simulink model "case6"  (R2024b)
settings: Solver=FixedStepAuto  StartTime=0  StopTime=1  FixedStep=1e-7  RelTol=1e-3
values from neighbouring files (symbols this model uses):
  SG_D_1_D = 0.01056    [IEEE9_case_parameters.m]    (also in case1_parameters.m; case2_parameters.m; case3_parameters.m; case4_parameters.m)
  SG_D_1_EnableSaturation = 0    [IEEE9_case_parameters.m]    (also in case1_parameters.m; case2_parameters.m; case3_parameters.m; case4_parameters.m)
  SG_D_1_f0 = 60    [IEEE9_case_parameters.m]    (also in case1_parameters.m; case2_parameters.m; case3_parameters.m; case4_parameters.m)
  SG_D_1_H = 7.5    [IEEE9_case_parameters.m]    (also in case1_parameters.m; case2_parameters.m; case3_parameters.m; case4_parameters.m)
  SG_D_1_K_A = 20    [IEEE9_case_parameters.m]    (also in case1_parameters.m; case2_parameters.m; case3_parameters.m; case4_parameters.m)
  SG_D_1_K_E = 1.000000e+1    (= 10)    [IEEE9_case_parameters.m]    (also in case1_parameters.m; case2_parameters.m; case3_parameters.m; case4_parameters.m)
  SG_D_1_K_F = 2.363    [IEEE9_case_parameters.m]    (also in case1_parameters.m; case2_parameters.m; case3_parameters.m; case4_parameters.m)
  SG_D_1_K_s = 0.5    [IEEE9_case_parameters.m]    (also in case1_parameters.m = 5; case2_parameters.m = 5; case3_parameters.m = 5; case4_parameters.m = 5)
  SG_D_1_R_a = 0.001088    [IEEE9_case_parameters.m]    (also in case1_parameters.m; case2_parameters.m; case3_parameters.m; case4_parameters.m)
  SG_D_1_S_A = 1    [IEEE9_case_parameters.m]    (also in case1_parameters.m; case2_parameters.m; case3_parameters.m; case4_parameters.m)
  SG_D_1_S_B = 0.103    [IEEE9_case_parameters.m]    (also in case1_parameters.m; case2_parameters.m; case3_parameters.m; case4_parameters.m)
  SG_D_1_S_N = 10.659857    [IEEE9_case_parameters.m]    (also in case1_parameters.m; case2_parameters.m; case3_parameters.m; case4_parameters.m)
  SG_D_1_SpeedPara = 200    [IEEE9_case_parameters.m]    (also in case1_parameters.m; case2_parameters.m; case3_parameters.m; case4_parameters.m)
  SG_D_1_T_0 = 0.720173    [IEEE9_case_parameters.m]    (also in case1_parameters.m = 0.755522; case2_parameters.m = 0.808931; case3_parameters.m = 0.869402; case4_parameters.m = 0.729316)
  SG_D_1_T_1 = 0.3    [IEEE9_case_parameters.m]    (also in case1_parameters.m; case2_parameters.m; case3_parameters.m; case4_parameters.m)
  SG_D_1_T_2 = 0.05    [IEEE9_case_parameters.m]    (also in case1_parameters.m; case2_parameters.m; case3_parameters.m; case4_parameters.m)
  SG_D_1_T_3 = 0.02    [IEEE9_case_parameters.m]    (also in case1_parameters.m; case2_parameters.m; case3_parameters.m; case4_parameters.m)
  SG_D_1_T_4 = 0.005    [IEEE9_case_parameters.m]    (also in case1_parameters.m; case2_parameters.m; case3_parameters.m; case4_parameters.m)
  SG_D_1_T_A = 0.02    [IEEE9_case_parameters.m]    (also in case1_parameters.m; case2_parameters.m; case3_parameters.m; case4_parameters.m)
  SG_D_1_T_dd = 8.000000e+0    (= 8)    [IEEE9_case_parameters.m]    (also in case1_parameters.m; case2_parameters.m; case3_parameters.m; case4_parameters.m)
  SG_D_1_T_ddd = 0.04    [IEEE9_case_parameters.m]    (also in case1_parameters.m; case2_parameters.m; case3_parameters.m; case4_parameters.m)
  SG_D_1_T_E = 0.314    [IEEE9_case_parameters.m]    (also in case1_parameters.m; case2_parameters.m; case3_parameters.m; case4_parameters.m)
  SG_D_1_T_F = 0.35    [IEEE9_case_parameters.m]    (also in case1_parameters.m; case2_parameters.m; case3_parameters.m; case4_parameters.m)
  SG_D_1_T_qd = 0.8    [IEEE9_case_parameters.m]    (also in case1_parameters.m; case2_parameters.m; case3_parameters.m; case4_parameters.m)
  SG_D_1_T_qdd = 0.02    [IEEE9_case_parameters.m]    (also in case1_parameters.m; case2_parameters.m; case3_parameters.m; case4_parameters.m)
  SG_D_1_T_speed = 0.1    [IEEE9_case_parameters.m]    (also in case1_parameters.m = 200; case2_parameters.m = 200; case3_parameters.m = 200; case4_parameters.m = 200)
  SG_D_1_T_w = 0.5    [IEEE9_case_parameters.m]    (also in case1_parameters.m; case2_parameters.m; case3_parameters.m; case4_parameters.m)
  SG_D_1_V_ref = 1.990276    [IEEE9_case_parameters.m]    (also in case1_parameters.m = 2.042296; case2_parameters.m = 2.051388; case3_parameters.m = 2.089584; case4_parameters.m = 2.01845)
  SG_D_1_w_ref = 376.991118    [IEEE9_case_parameters.m]    (also in case1_parameters.m; case2_parameters.m; case3_parameters.m; case4_parameters.m)
  SG_D_1_wb = 6.000000e+1    (= 60)    [IEEE9_case_parameters.m]    (also in case1_parameters.m; case2_parameters.m; case3_parameters.m; case4_parameters.m)
  SG_D_1_x_d = 1.9    [IEEE9_case_parameters.m]    (also in case1_parameters.m; case2_parameters.m; case3_parameters.m; case4_parameters.m)
  SG_D_1_x_dd = 0.302    [IEEE9_case_parameters.m]    (also in case1_parameters.m; case2_parameters.m; case3_parameters.m; case4_parameters.m)
  SG_D_1_x_ddd = 0.204    [IEEE9_case_parameters.m]    (also in case1_parameters.m; case2_parameters.m; case3_parameters.m; case4_parameters.m)
  SG_D_1_x_l = 0.05    [IEEE9_case_parameters.m]    (also in case1_parameters.m; case2_parameters.m; case3_parameters.m; case4_parameters.m)
  SG_D_1_x_q = 1.3    [IEEE9_case_parameters.m]    (also in case1_parameters.m; case2_parameters.m; case3_parameters.m; case4_parameters.m)
  SG_D_1_x_qd = 0.5    [IEEE9_case_parameters.m]    (also in case1_parameters.m; case2_parameters.m; case3_parameters.m; case4_parameters.m)
  SG_D_1_x_qdd = 0.3    [IEEE9_case_parameters.m]    (also in case1_parameters.m; case2_parameters.m; case3_parameters.m; case4_parameters.m)
  SG_D_2_D = 0.02    [IEEE9_case_parameters.m]    (also in case1_parameters.m; case2_parameters.m; case3_parameters.m; case4_parameters.m)
  SG_D_2_EnableSaturation = 0    [IEEE9_case_parameters.m]    (also in case1_parameters.m; case2_parameters.m; case3_parameters.m; case4_parameters.m)
  SG_D_2_f0 = 60    [IEEE9_case_parameters.m]    (also in case1_parameters.m; case2_parameters.m; case3_parameters.m; case4_parameters.m)
  SG_D_2_H = 8.000000e+0    (= 8)    [IEEE9_case_parameters.m]    (also in case1_parameters.m; case2_parameters.m; case3_parameters.m; case4_parameters.m)
  SG_D_2_K_A = 20    [IEEE9_case_parameters.m]    (also in case1_parameters.m; case2_parameters.m; case3_parameters.m; case4_parameters.m)
  SG_D_2_K_E = 1.000000e+1    (= 10)    [IEEE9_case_parameters.m]    (also in case1_parameters.m; case2_parameters.m; case3_parameters.m; case4_parameters.m)
  SG_D_2_K_F = 2.363    [IEEE9_case_parameters.m]    (also in case1_parameters.m; case2_parameters.m; case3_parameters.m; case4_parameters.m)
  SG_D_2_K_s = 0.5    [IEEE9_case_parameters.m]    (also in case1_parameters.m = 4; case2_parameters.m = 4; case3_parameters.m = 4; case4_parameters.m = 4)
  SG_D_2_R_a = 0.001088    [IEEE9_case_parameters.m]    (also in case1_parameters.m; case2_parameters.m; case3_parameters.m; case4_parameters.m)
  SG_D_2_S_A = 1    [IEEE9_case_parameters.m]    (also in case1_parameters.m; case2_parameters.m; case3_parameters.m; case4_parameters.m)
  SG_D_2_S_B = 0.103    [IEEE9_case_parameters.m]    (also in case1_parameters.m; case2_parameters.m; case3_parameters.m; case4_parameters.m)
  SG_D_2_S_N = 10.659857    [IEEE9_case_parameters.m]    (also in case1_parameters.m; case2_parameters.m; case3_parameters.m; case4_parameters.m)
  SG_D_2_SpeedPara = 200    [IEEE9_case_parameters.m]    (also in case1_parameters.m; case2_parameters.m; case3_parameters.m; case4_parameters.m)
  SG_D_2_T_0 = 1.632913    [IEEE9_case_parameters.m]    (also in case1_parameters.m = 1.632925; case2_parameters.m = 1.632915; case3_parameters.m = 1.632914; case4_parameters.m = 1.632927)
  SG_D_2_T_1 = 0.2    [IEEE9_case_parameters.m]    (also in case1_parameters.m; case2_parameters.m; case3_parameters.m; case4_parameters.m)
  SG_D_2_T_2 = 0.05    [IEEE9_case_parameters.m]    (also in case1_parameters.m; case2_parameters.m; case3_parameters.m; case4_parameters.m)
  SG_D_2_T_3 = 0.02    [IEEE9_case_parameters.m]    (also in case1_parameters.m; case2_parameters.m; case3_parameters.m; case4_parameters.m)
  SG_D_2_T_4 = 0.005    [IEEE9_case_parameters.m]    (also in case1_parameters.m; case2_parameters.m; case3_parameters.m; case4_parameters.m)
  SG_D_2_T_A = 0.02    [IEEE9_case_parameters.m]    (also in case1_parameters.m; case2_parameters.m; case3_parameters.m; case4_parameters.m)
  SG_D_2_T_dd = 7.9    [IEEE9_case_parameters.m]    (also in case1_parameters.m; case2_parameters.m; case3_parameters.m; case4_parameters.m)
  SG_D_2_T_ddd = 0.04    [IEEE9_case_parameters.m]    (also in case1_parameters.m; case2_parameters.m; case3_parameters.m; case4_parameters.m)
  SG_D_2_T_E = 0.314    [IEEE9_case_parameters.m]    (also in case1_parameters.m; case2_parameters.m; case3_parameters.m; case4_parameters.m)
  SG_D_2_T_F = 0.35    [IEEE9_case_parameters.m]    (also in case1_parameters.m; case2_parameters.m; case3_parameters.m; case4_parameters.m)
  SG_D_2_T_qd = 0.8    [IEEE9_case_parameters.m]    (also in case1_parameters.m; case2_parameters.m; case3_parameters.m; case4_parameters.m)
  SG_D_2_T_qdd = 0.015    [IEEE9_case_parameters.m]    (also in case1_parameters.m; case2_parameters.m; case3_parameters.m; case4_parameters.m)
  SG_D_2_T_speed = 0.1    [IEEE9_case_parameters.m]    (also in case1_parameters.m = 150; case2_parameters.m = 150; case3_parameters.m = 150; case4_parameters.m = 150)
  SG_D_2_T_w = 0.35    [IEEE9_case_parameters.m]    (also in case1_parameters.m; case2_parameters.m; case3_parameters.m; case4_parameters.m)
  SG_D_2_V_ref = 2.58547    [IEEE9_case_parameters.m]    (also in case1_parameters.m = 2.597896; case2_parameters.m = 2.587136; case3_parameters.m = 2.586042; case4_parameters.m = 2.599679)
  SG_D_2_w_ref = 376.991118    [IEEE9_case_parameters.m]    (also in case1_parameters.m; case2_parameters.m; case3_parameters.m; case4_parameters.m)
  SG_D_2_wb = 6.000000e+1    (= 60)    [IEEE9_case_parameters.m]    (also in case1_parameters.m; case2_parameters.m; case3_parameters.m; case4_parameters.m)
  SG_D_2_x_d = 1.8    [IEEE9_case_parameters.m]    (also in case1_parameters.m; case2_parameters.m; case3_parameters.m; case4_parameters.m)
  SG_D_2_x_dd = 0.302    [IEEE9_case_parameters.m]    (also in case1_parameters.m; case2_parameters.m; case3_parameters.m; case4_parameters.m)
  SG_D_2_x_ddd = 0.204    [IEEE9_case_parameters.m]    (also in case1_parameters.m; case2_parameters.m; case3_parameters.m; case4_parameters.m)
  SG_D_2_x_l = 0.05    [IEEE9_case_parameters.m]    (also in case1_parameters.m; case2_parameters.m; case3_parameters.m; case4_parameters.m)
  SG_D_2_x_q = 1.25    [IEEE9_case_parameters.m]    (also in case1_parameters.m; case2_parameters.m; case3_parameters.m; case4_parameters.m)
  SG_D_2_x_qd = 0.5    [IEEE9_case_parameters.m]    (also in case1_parameters.m; case2_parameters.m; case3_parameters.m; case4_parameters.m)
  SG_D_2_x_qdd = 0.3    [IEEE9_case_parameters.m]    (also in case1_parameters.m; case2_parameters.m; case3_parameters.m; case4_parameters.m)
  SG_D_3_D = 0.02    [IEEE9_case_parameters.m]    (also in case1_parameters.m; case2_parameters.m; case3_parameters.m; case4_parameters.m)
  SG_D_3_EnableSaturation = 0    [IEEE9_case_parameters.m]    (also in case1_parameters.m; case2_parameters.m; case3_parameters.m; case4_parameters.m)
  SG_D_3_f0 = 60    [IEEE9_case_parameters.m]    (also in case1_parameters.m; case2_parameters.m; case3_parameters.m; case4_parameters.m)
  SG_D_3_H = 7.7    [IEEE9_case_parameters.m]    (also in case1_parameters.m; case2_parameters.m; case3_parameters.m; case4_parameters.m)
  SG_D_3_K_A = 20    [IEEE9_case_parameters.m]    (also in case1_parameters.m; case2_parameters.m; case3_parameters.m; case4_parameters.m)
  SG_D_3_K_E = 1.000000e+1    (= 10)    [IEEE9_case_parameters.m]    (also in case1_parameters.m; case2_parameters.m; case3_parameters.m; case4_parameters.m)
  SG_D_3_K_F = 2.363    [IEEE9_case_parameters.m]    (also in case1_parameters.m; case2_parameters.m; case3_parameters.m; case4_parameters.m)
  SG_D_3_K_s = 0.2    [IEEE9_case_parameters.m]    (also in case1_parameters.m = 2; case2_parameters.m = 2; case3_parameters.m = 2; case4_parameters.m = 2)
  SG_D_3_R_a = 0.001088    [IEEE9_case_parameters.m]    (also in case1_parameters.m; case2_parameters.m; case3_parameters.m; case4_parameters.m)
  SG_D_3_S_A = 1    [IEEE9_case_parameters.m]    (also in case1_parameters.m; case2_parameters.m; case3_parameters.m; case4_parameters.m)
  SG_D_3_S_B = 0.103    [IEEE9_case_parameters.m]    (also in case1_parameters.m; case2_parameters.m; case3_parameters.m; case4_parameters.m)
  SG_D_3_S_N = 10.659857    [IEEE9_case_parameters.m]    (also in case1_parameters.m; case2_parameters.m; case3_parameters.m; case4_parameters.m)
  SG_D_3_SpeedPara = 200    [IEEE9_case_parameters.m]    (also in case1_parameters.m; case2_parameters.m; case3_parameters.m; case4_parameters.m)
  SG_D_3_T_0 = 0.850788    [IEEE9_case_parameters.m]    (also in case1_parameters.m = 0.850786; case2_parameters.m = 0.850787; case3_parameters.m; case4_parameters.m = 0.850786)
  SG_D_3_T_1 = 0.2    [IEEE9_case_parameters.m]    (also in case1_parameters.m; case2_parameters.m; case3_parameters.m; case4_parameters.m)
  SG_D_3_T_2 = 0.05    [IEEE9_case_parameters.m]    (also in case1_parameters.m; case2_parameters.m; case3_parameters.m; case4_parameters.m)
  SG_D_3_T_3 = 0.02    [IEEE9_case_parameters.m]    (also in case1_parameters.m; case2_parameters.m; case3_parameters.m; case4_parameters.m)
  SG_D_3_T_4 = 0.005    [IEEE9_case_parameters.m]    (also in case1_parameters.m; case2_parameters.m; case3_parameters.m; case4_parameters.m)
  SG_D_3_T_A = 0.02    [IEEE9_case_parameters.m]    (also in case1_parameters.m; case2_parameters.m; case3_parameters.m; case4_parameters.m)
  SG_D_3_T_dd = 8.1    [IEEE9_case_parameters.m]    (also in case1_parameters.m; case2_parameters.m; case3_parameters.m; case4_parameters.m)
  SG_D_3_T_ddd = 0.04    [IEEE9_case_parameters.m]    (also in case1_parameters.m; case2_parameters.m; case3_parameters.m; case4_parameters.m)
  SG_D_3_T_E = 0.314    [IEEE9_case_parameters.m]    (also in case1_parameters.m; case2_parameters.m; case3_parameters.m; case4_parameters.m)
  SG_D_3_T_F = 0.35    [IEEE9_case_parameters.m]    (also in case1_parameters.m; case2_parameters.m; case3_parameters.m; case4_parameters.m)
  SG_D_3_T_qd = 0.8    [IEEE9_case_parameters.m]    (also in case1_parameters.m; case2_parameters.m; case3_parameters.m; case4_parameters.m)
  SG_D_3_T_qdd = 0.015    [IEEE9_case_parameters.m]    (also in case1_parameters.m; case2_parameters.m; case3_parameters.m; case4_parameters.m)
  SG_D_3_T_speed = 0.1    [IEEE9_case_parameters.m]    (also in case1_parameters.m = 180; case2_parameters.m = 180; case3_parameters.m = 180; case4_parameters.m = 180)
  SG_D_3_T_w = 0.4    [IEEE9_case_parameters.m]    (also in case1_parameters.m; case2_parameters.m; case3_parameters.m; case4_parameters.m)
  SG_D_3_V_ref = 1.892727    [IEEE9_case_parameters.m]    (also in case1_parameters.m = 1.906439; case2_parameters.m = 1.895535; case3_parameters.m = 1.892105; case4_parameters.m = 1.906598)
  SG_D_3_w_ref = 376.991118    [IEEE9_case_parameters.m]    (also in case1_parameters.m; case2_parameters.m; case3_parameters.m; case4_parameters.m)
  SG_D_3_wb = 6.000000e+1    (= 60)    [IEEE9_case_parameters.m]    (also in case1_parameters.m; case2_parameters.m; case3_parameters.m; case4_parameters.m)
  SG_D_3_x_d = 1.85    [IEEE9_case_parameters.m]    (also in case1_parameters.m; case2_parameters.m; case3_parameters.m; case4_parameters.m)
  SG_D_3_x_dd = 0.302    [IEEE9_case_parameters.m]    (also in case1_parameters.m; case2_parameters.m; case3_parameters.m; case4_parameters.m)
  SG_D_3_x_ddd = 0.204    [IEEE9_case_parameters.m]    (also in case1_parameters.m; case2_parameters.m; case3_parameters.m; case4_parameters.m)
  SG_D_3_x_l = 0.05    [IEEE9_case_parameters.m]    (also in case1_parameters.m; case2_parameters.m; case3_parameters.m; case4_parameters.m)
  SG_D_3_x_q = 1.2    [IEEE9_case_parameters.m]    (also in case1_parameters.m; case2_parameters.m; case3_parameters.m; case4_parameters.m)
  SG_D_3_x_qd = 0.5    [IEEE9_case_parameters.m]    (also in case1_parameters.m; case2_parameters.m; case3_parameters.m; case4_parameters.m)
  SG_D_3_x_qdd = 0.3    [IEEE9_case_parameters.m]    (also in case1_parameters.m; case2_parameters.m; case3_parameters.m; case4_parameters.m)
(part 3 of 12)

== system case6/AC_1/d_id_load_7_block ==
  note: d_id_load_7 in case6
      | $376.991118430775\,\mathrm{iq}_{\mathrm{load},7}-1042.68025815291\,\mathrm{id}_{\mathrm{load},7}+1171.3449213978\,\mathrm{vd}_{\mathrm{bus},7}$
      | Automatically generated on 2025-10-31 19:20:41 .
  State_id_load_7_ed6d0 : Inport
  State_iq_load_7_25236 : Inport  Port=2
  State_vd_bus_7_f8e0f : Inport  Port=3
  Add_24cd1 : Sum
  Add_83972 : Sum
  Constant_-1042.68025815291_f7e22 : Constant  Value=-1042.68025815291
  Constant_1171.3449213978_b1cfa : Constant  Value=1171.3449213978
  Constant_376.991118430775_13427 : Constant  Value=376.991118430775
  Product_2e9ca : Product
  Product_abc47 : Product
  Product_b8994 : Product
  Blockout_d_id_load_7_4bf44 : Outport
  wires:
  Constant_-1042.68025815291_f7e22/1 -> Product_2e9ca/1
  Product_b8994/1 -> Add_83972/2
  State_id_load_7_ed6d0/1 -> Product_2e9ca/2
  Constant_376.991118430775_13427/1 -> Product_b8994/1
  Product_2e9ca/1 -> Add_83972/1
  State_iq_load_7_25236/1 -> Product_b8994/2
  Constant_1171.3449213978_b1cfa/1 -> Product_abc47/1
  State_vd_bus_7_f8e0f/1 -> Product_abc47/2
  Add_83972/1 -> Add_24cd1/1
  Product_abc47/1 -> Add_24cd1/2
  Add_24cd1/1 -> Blockout_d_id_load_7_4bf44/1

== system case6/AC_1/d_id_load_9_block ==
  note: d_id_load_9 in case6
      | $376.991118430775\,\mathrm{iq}_{\mathrm{load},9}-912.345225962008\,\mathrm{id}_{\mathrm{load},9}+1407.02236836831\,\mathrm{vd}_{\mathrm{bus},9}$
      | Automatically generated on 2025-10-31 19:20:44 .
  State_id_load_9_971b0 : Inport
  State_iq_load_9_63cda : Inport  Port=2
  State_vd_bus_9_1fdd2 : Inport  Port=3
  Add_11f24 : Sum
  Add_b37a4 : Sum
  Constant_-912.345225962008_b413d : Constant  Value=-912.345225962008
  Constant_1407.02236836831_5bcda : Constant  Value=1407.02236836831
  Constant_376.991118430775_b0d4f : Constant  Value=376.991118430775
  Product_84c17 : Product
  Product_90090 : Product
  Product_fc741 : Product
  Blockout_d_id_load_9_0a7d1 : Outport
  wires:
  Constant_-912.345225962008_b413d/1 -> Product_84c17/1
  Product_90090/1 -> Add_b37a4/2
  State_id_load_9_971b0/1 -> Product_84c17/2
  Constant_376.991118430775_b0d4f/1 -> Product_90090/1
  Product_84c17/1 -> Add_b37a4/1
  State_iq_load_9_63cda/1 -> Product_90090/2
  Constant_1407.02236836831_5bcda/1 -> Product_fc741/1
  State_vd_bus_9_1fdd2/1 -> Product_fc741/2
  Add_b37a4/1 -> Add_11f24/1
  Product_fc741/1 -> Add_11f24/2
  Add_11f24/1 -> Blockout_d_id_load_9_0a7d1/1

== system case6/AC_1/d_iq_line_1_4_block ==
  note: d_iq_line_1_4 in case6
      | $6868.34433494245\,\mathrm{vq}_{\mathrm{bus},1}-376.991118430775\,\mathrm{id}_{\mathrm{line},1,4}-6868.34433494245\,\mathrm{vq}_{\mathrm{bus},4}$
      | Automatically generated on 2025-10-31 19:20:48 .
  State_id_line_1_4_5a9b1 : Inport
  State_vq_bus_1_6b284 : Inport  Port=2
  State_vq_bus_4_deba6 : Inport  Port=3
  Add_c85ec : Sum
  Constant_-376.991118430775_bb66e : Constant  Value=-376.991118430775
  Constant_6868.34433494245_3906b : Constant  Value=6868.34433494245
  Constant_6868.34433494245_64567 : Constant  Value=6868.34433494245
  Product_0c770 : Product
  Product_838f3 : Product
  Product_8e35f : Product
  Subtract_df51f : Sum  Inputs=+-
  Blockout_d_iq_line_1_4_201af : Outport
  wires:
  Constant_-376.991118430775_bb66e/1 -> Product_0c770/1
  Product_8e35f/1 -> Add_c85ec/2
  State_id_line_1_4_5a9b1/1 -> Product_0c770/2
  Constant_6868.34433494245_3906b/1 -> Product_8e35f/1
  Product_0c770/1 -> Add_c85ec/1
  Subtract_df51f/1 -> Blockout_d_iq_line_1_4_201af/1
  State_vq_bus_1_6b284/1 -> Product_8e35f/2
  Constant_6868.34433494245_64567/1 -> Product_838f3/1
  State_vq_bus_4_deba6/1 -> Product_838f3/2
  Add_c85ec/1 -> Subtract_df51f/1
  Product_838f3/1 -> Subtract_df51f/2

== system case6/AC_1/d_iq_line_3_6_block ==
  note: d_iq_line_3_6 in case6
      | $6751.13709373183\,\mathrm{vq}_{\mathrm{bus},3}-376.991118430775\,\mathrm{id}_{\mathrm{line},3,6}-6751.13709373183\,\mathrm{vq}_{\mathrm{bus},6}$
      | Automatically generated on 2025-10-31 19:20:58 .
  State_id_line_3_6_29fbd : Inport
  State_vq_bus_3_8aa9d : Inport  Port=2
  State_vq_bus_6_e5847 : Inport  Port=3
  Add_bc3ba : Sum
  Constant_-376.991118430775_cf978 : Constant  Value=-376.991118430775
  Constant_6751.13709373183_457c0 : Constant  Value=6751.13709373183
  Constant_6751.13709373183_acfcf : Constant  Value=6751.13709373183
  Product_533ae : Product
  Product_6e6cb : Product
  Product_998dd : Product
  Subtract_d0816 : Sum  Inputs=+-
  Blockout_d_iq_line_3_6_a81a1 : Outport
  wires:
  Constant_-376.991118430775_cf978/1 -> Product_533ae/1
  Product_6e6cb/1 -> Add_bc3ba/2
  State_id_line_3_6_29fbd/1 -> Product_533ae/2
  Constant_6751.13709373183_acfcf/1 -> Product_6e6cb/1
  Product_533ae/1 -> Add_bc3ba/1
  State_vq_bus_3_8aa9d/1 -> Product_6e6cb/2
  Constant_6751.13709373183_457c0/1 -> Product_998dd/1
  State_vq_bus_6_e5847/1 -> Product_998dd/2
  Add_bc3ba/1 -> Subtract_d0816/1
  Product_998dd/1 -> Subtract_d0816/2
  Subtract_d0816/1 -> Blockout_d_iq_line_3_6_a81a1/1

== system case6/AC_1/d_iq_line_4_5_block ==
  note: d_iq_line_4_5 in case6
      | $4300.18080100745\,\mathrm{vq}_{\mathrm{bus},4}-80.0510363901558\,\mathrm{iq}_{\mathrm{line},4,5}-376.991118430775\,\mathrm{id}_{\mathrm{line},4,5}-4300.18080100745\,\mathrm{vq}_{\mathrm{bus},5}$
      | Automatically generated on 2025-10-31 19:20:51 .
  State_id_line_4_5_745b5 : Inport
  State_iq_line_4_5_ac887 : Inport  Port=2
  State_vq_bus_4_3ba67 : Inport  Port=3
  State_vq_bus_5_1f302 : Inport  Port=4
  Add_3f9cb : Sum
  Constant_-376.991118430775_905c7 : Constant  Value=-376.991118430775
  Constant_4300.18080100745_5ac1a : Constant  Value=4300.18080100745
  Constant_4300.18080100745_dda01 : Constant  Value=4300.18080100745
  Constant_80.0510363901558_07483 : Constant  Value=80.0510363901558
  Product_63045 : Product
  Product_696cc : Product
  Product_76f35 : Product
  Product_a9744 : Product
  Subtract_069a5 : Sum  Inputs=+-
  Subtract_aa349 : Sum  Inputs=+-
  Blockout_d_iq_line_4_5_20bf0 : Outport
  wires:
  Constant_-376.991118430775_905c7/1 -> Product_696cc/1
  Constant_80.0510363901558_07483/1 -> Product_63045/1
  State_id_line_4_5_745b5/1 -> Product_696cc/2
  State_iq_line_4_5_ac887/1 -> Product_63045/2
  Product_696cc/1 -> Subtract_069a5/1
  Constant_4300.18080100745_dda01/1 -> Product_76f35/1
  Product_63045/1 -> Subtract_069a5/2
  State_vq_bus_4_3ba67/1 -> Product_76f35/2
  Subtract_069a5/1 -> Add_3f9cb/1
  Product_76f35/1 -> Add_3f9cb/2
  Constant_4300.18080100745_5ac1a/1 -> Product_a9744/1
  State_vq_bus_5_1f302/1 -> Product_a9744/2
  Add_3f9cb/1 -> Subtract_aa349/1
  Product_a9744/1 -> Subtract_aa349/2
  Subtract_aa349/1 -> Blockout_d_iq_line_4_5_20bf0/1

== system case6/AC_1/d_iq_line_5_6_block ==
  note: d_iq_line_5_6 in case6
      | $2327.1566687805\,\mathrm{vq}_{\mathrm{bus},5}-99.3851621342142\,\mathrm{iq}_{\mathrm{line},5,6}-376.991118430775\,\mathrm{id}_{\mathrm{line},5,6}-2327.1566687805\,\mathrm{vq}_{\mathrm{bus},6}$
      | Automatically generated on 2025-10-31 19:20:55 .
  State_id_line_5_6_ed5dc : Inport
  State_iq_line_5_6_5beea : Inport  Port=2
  State_vq_bus_5_fd8ff : Inport  Port=3
  State_vq_bus_6_9dc1c : Inport  Port=4
  Add_794ba : Sum
  Constant_-376.991118430775_0cdd4 : Constant  Value=-376.991118430775
  Constant_2327.1566687805_6204d : Constant  Value=2327.1566687805
  Constant_2327.1566687805_ecfc1 : Constant  Value=2327.1566687805
  Constant_99.3851621342142_77585 : Constant  Value=99.3851621342142
  Product_0c66e : Product
  Product_0e0ca : Product
  Product_342fd : Product
  Product_52106 : Product
  Subtract_0c098 : Sum  Inputs=+-
  Subtract_67df0 : Sum  Inputs=+-
  Blockout_d_iq_line_5_6_a7a19 : Outport
  wires:
  Constant_-376.991118430775_0cdd4/1 -> Product_0c66e/1
  Constant_99.3851621342142_77585/1 -> Product_342fd/1
  Subtract_0c098/1 -> Blockout_d_iq_line_5_6_a7a19/1
  State_id_line_5_6_ed5dc/1 -> Product_0c66e/2
  State_iq_line_5_6_5beea/1 -> Product_342fd/2
  Product_0c66e/1 -> Subtract_67df0/1
  Constant_2327.1566687805_6204d/1 -> Product_52106/1
  Product_342fd/1 -> Subtract_67df0/2
  Product_0e0ca/1 -> Subtract_0c098/2
  State_vq_bus_5_fd8ff/1 -> Product_52106/2
  Subtract_67df0/1 -> Add_794ba/1
  Product_52106/1 -> Add_794ba/2
  Constant_2327.1566687805_ecfc1/1 -> Product_0e0ca/1
  State_vq_bus_6_9dc1c/1 -> Product_0e0ca/2
  Add_794ba/1 -> Subtract_0c098/1

== system case6/AC_1/d_iq_line_6_7_block ==
  note: d_iq_line_6_7 in case6
      | $3924.76819139569\,\mathrm{vq}_{\mathrm{bus},6}-51.1437176937107\,\mathrm{iq}_{\mathrm{line},6,7}-376.991118430775\,\mathrm{id}_{\mathrm{line},6,7}-3924.76819139569\,\mathrm{vq}_{\mathrm{bus},7}$
      | Automatically generated on 2025-10-31 19:21:01 .
  State_id_line_6_7_b680f : Inport
  State_iq_line_6_7_4945e : Inport  Port=2
  State_vq_bus_6_e12d0 : Inport  Port=3
  State_vq_bus_7_e72a8 : Inport  Port=4
  Add_53d93 : Sum
  Constant_-376.991118430775_8e837 : Constant  Value=-376.991118430775
  Constant_3924.76819139569_0230c : Constant  Value=3924.76819139569
  Constant_3924.76819139569_cdb64 : Constant  Value=3924.76819139569
  Constant_51.1437176937107_d8d9f : Constant  Value=51.1437176937107
  Product_22186 : Product
  Product_3b982 : Product
  Product_6a558 : Product
  Product_832d5 : Product
  Subtract_028f3 : Sum  Inputs=+-
  Subtract_95e0c : Sum  Inputs=+-
  Blockout_d_iq_line_6_7_9a304 : Outport
  wires:
  Constant_-376.991118430775_8e837/1 -> Product_22186/1
  Constant_51.1437176937107_d8d9f/1 -> Product_832d5/1
  State_id_line_6_7_b680f/1 -> Product_22186/2
  State_iq_line_6_7_4945e/1 -> Product_832d5/2
  Product_22186/1 -> Subtract_028f3/1
  Constant_3924.76819139569_0230c/1 -> Product_3b982/1
  Product_832d5/1 -> Subtract_028f3/2
  State_vq_bus_6_e12d0/1 -> Product_3b982/2
  Subtract_028f3/1 -> Add_53d93/1
  Product_3b982/1 -> Add_53d93/2
  Constant_3924.76819139569_cdb64/1 -> Product_6a558/1
  State_vq_bus_7_e72a8/1 -> Product_6a558/2
  Add_53d93/1 -> Subtract_95e0c/1
  Product_6a558/1 -> Subtract_95e0c/2
  Subtract_95e0c/1 -> Blockout_d_iq_line_6_7_9a304/1

== system case6/AC_1/d_iq_line_7_8_block ==
  note: d_iq_line_7_8 in case6
      | $5494.67546795396\,\mathrm{vq}_{\mathrm{bus},7}-51.1437176937107\,\mathrm{iq}_{\mathrm{line},7,8}-376.991118430775\,\mathrm{id}_{\mathrm{line},7,8}-5494.67546795396\,\mathrm{vq}_{\mathrm{bus},8}$
      | Automatically generated on 2025-10-31 19:21:05 .
  State_id_line_7_8_93183 : Inport
  State_iq_line_7_8_31614 : Inport  Port=2
  State_vq_bus_7_c9505 : Inport  Port=3
  State_vq_bus_8_642dd : Inport  Port=4
  Add_d027a : Sum
  Constant_-376.991118430775_0ce04 : Constant  Value=-376.991118430775
  Constant_51.1437176937107_c8d26 : Constant  Value=51.1437176937107
  Constant_5494.67546795396_683a1 : Constant  Value=5494.67546795396
  Constant_5494.67546795396_aa560 : Constant  Value=5494.67546795396
  Product_9cf54 : Product
  Product_9f72a : Product
  Product_ee26a : Product
  Product_f6aa3 : Product
  Subtract_c1d3c : Sum  Inputs=+-
  Subtract_ecd13 : Sum  Inputs=+-
  Blockout_d_iq_line_7_8_31fbf : Outport
  wires:
  Constant_-376.991118430775_0ce04/1 -> Product_f6aa3/1
  Constant_51.1437176937107_c8d26/1 -> Product_9cf54/1
  State_id_line_7_8_93183/1 -> Product_f6aa3/2
  State_iq_line_7_8_31614/1 -> Product_9cf54/2
  Product_f6aa3/1 -> Subtract_c1d3c/1
  Constant_5494.67546795396_683a1/1 -> Product_9f72a/1
  Product_9cf54/1 -> Subtract_c1d3c/2
  State_vq_bus_7_c9505/1 -> Product_9f72a/2
  Subtract_c1d3c/1 -> Add_d027a/1
  Product_9f72a/1 -> Add_d027a/2
  Constant_5494.67546795396_aa560/1 -> Product_ee26a/1
  State_vq_bus_8_642dd/1 -> Product_ee26a/2
  Add_d027a/1 -> Subtract_ecd13/1
  Product_ee26a/1 -> Subtract_ecd13/2
  Subtract_ecd13/1 -> Blockout_d_iq_line_7_8_31fbf/1

== system case6/AC_1/d_iq_line_8_2_block ==
  note: d_iq_line_8_2 in case6
      | $6329.86613908296\,\mathrm{vq}_{\mathrm{bus},8}-6329.86613908296\,\mathrm{vq}_{\mathrm{bus},2}-376.991118430775\,\mathrm{id}_{\mathrm{line},8,2}$
      | Automatically generated on 2025-10-31 19:21:07 .
  State_id_line_8_2_11e9c : Inport
  State_vq_bus_2_4380d : Inport  Port=2
  State_vq_bus_8_42f30 : Inport  Port=3
  Add_87672 : Sum
  Constant_-376.991118430775_38a13 : Constant  Value=-376.991118430775
  Constant_6329.86613908296_3f223 : Constant  Value=6329.86613908296
  Constant_6329.86613908296_b3b66 : Constant  Value=6329.86613908296
  Product_022d2 : Product
  Product_34368 : Product
  Product_4c8f7 : Product
  Subtract_34b41 : Sum  Inputs=+-
  Blockout_d_iq_line_8_2_47ccc : Outport
  wires:
  Constant_-376.991118430775_38a13/1 -> Product_022d2/1
  Product_4c8f7/1 -> Subtract_34b41/2
  State_id_line_8_2_11e9c/1 -> Product_022d2/2
  Constant_6329.86613908296_b3b66/1 -> Product_4c8f7/1
  Product_022d2/1 -> Subtract_34b41/1
  State_vq_bus_2_4380d/1 -> Product_4c8f7/2
  Constant_6329.86613908296_3f223/1 -> Product_34368/1
  State_vq_bus_8_42f30/1 -> Product_34368/2
  Subtract_34b41/1 -> Add_87672/1
  Product_34368/1 -> Add_87672/2
  Add_87672/1 -> Blockout_d_iq_line_8_2_47ccc/1

== system case6/AC_1/d_iq_line_8_9_block ==
  note: d_iq_line_8_9 in case6
      | $2457.24617200426\,\mathrm{vq}_{\mathrm{bus},8}-86.1053164532769\,\mathrm{iq}_{\mathrm{line},8,9}-376.991118430775\,\mathrm{id}_{\mathrm{line},8,9}-2457.24617200426\,\mathrm{vq}_{\mathrm{bus},9}$
      | Automatically generated on 2025-10-31 19:21:11 .
  State_id_line_8_9_f86eb : Inport
  State_iq_line_8_9_58567 : Inport  Port=2
  State_vq_bus_8_cf718 : Inport  Port=3
  State_vq_bus_9_b3e7a : Inport  Port=4
  Add_c01ba : Sum
  Constant_-376.991118430775_8291a : Constant  Value=-376.991118430775
  Constant_2457.24617200426_b60d8 : Constant  Value=2457.24617200426
  Constant_2457.24617200426_fbb27 : Constant  Value=2457.24617200426
  Constant_86.1053164532769_a32aa : Constant  Value=86.1053164532769
  Product_41230 : Product
  Product_71b14 : Product
  Product_7ae5c : Product
  Product_a6780 : Product
  Subtract_56151 : Sum  Inputs=+-
  Subtract_87b4a : Sum  Inputs=+-
  Blockout_d_iq_line_8_9_46de9 : Outport
  wires:
  Constant_-376.991118430775_8291a/1 -> Product_7ae5c/1
  Constant_86.1053164532769_a32aa/1 -> Product_71b14/1
  State_id_line_8_9_f86eb/1 -> Product_7ae5c/2
  State_iq_line_8_9_58567/1 -> Product_71b14/2
  Product_7ae5c/1 -> Subtract_56151/1
  Constant_2457.24617200426_fbb27/1 -> Product_a6780/1
  Product_71b14/1 -> Subtract_56151/2
  State_vq_bus_8_cf718/1 -> Product_a6780/2
  Subtract_56151/1 -> Add_c01ba/1
  Product_a6780/1 -> Add_c01ba/2
  Constant_2457.24617200426_b60d8/1 -> Product_41230/1
  Add_c01ba/1 -> Subtract_87b4a/1
  State_vq_bus_9_b3e7a/1 -> Product_41230/2
  Product_41230/1 -> Subtract_87b4a/2
  Subtract_87b4a/1 -> Blockout_d_iq_line_8_9_46de9/1

== system case6/AC_1/d_iq_line_9_4_block ==
  note: d_iq_line_9_4 in case6
      | $4654.313337561\,\mathrm{vq}_{\mathrm{bus},9}-50.9667498124176\,\mathrm{iq}_{\mathrm{line},9,4}-4654.313337561\,\mathrm{vq}_{\mathrm{bus},4}-376.991118430775\,\mathrm{id}_{\mathrm{line},9,4}$
      | Automatically generated on 2025-10-31 19:21:14 .
  State_id_line_9_4_3cff0 : Inport
  State_iq_line_9_4_21c4a : Inport  Port=2
  State_vq_bus_4_9b47a : Inport  Port=3
  State_vq_bus_9_c88b7 : Inport  Port=4
  Add_1f19f : Sum
  Constant_-376.991118430775_9142e : Constant  Value=-376.991118430775
  Constant_4654.313337561_63b12 : Constant  Value=4654.313337561
  Constant_4654.313337561_93558 : Constant  Value=4654.313337561
  Constant_50.9667498124176_ab34e : Constant  Value=50.9667498124176
  Product_57fd2 : Product
  Product_85700 : Product
  Product_b123e : Product
  Product_f526d : Product
  Subtract_42515 : Sum  Inputs=+-
  Subtract_46daa : Sum  Inputs=+-
  Blockout_d_iq_line_9_4_b362e : Outport
  wires:
  Constant_-376.991118430775_9142e/1 -> Product_57fd2/1
  Constant_50.9667498124176_ab34e/1 -> Product_b123e/1
  State_id_line_9_4_3cff0/1 -> Product_57fd2/2
  State_iq_line_9_4_21c4a/1 -> Product_b123e/2
  Product_57fd2/1 -> Subtract_46daa/1
  Constant_4654.313337561_93558/1 -> Product_85700/1
  Product_b123e/1 -> Subtract_46daa/2
  State_vq_bus_4_9b47a/1 -> Product_85700/2
  Subtract_46daa/1 -> Subtract_42515/1
  Product_85700/1 -> Subtract_42515/2
  Constant_4654.313337561_63b12/1 -> Product_f526d/1
  Add_1f19f/1 -> Blockout_d_iq_line_9_4_b362e/1
  State_vq_bus_9_c88b7/1 -> Product_f526d/2
  Subtract_42515/1 -> Add_1f19f/1
  Product_f526d/1 -> Add_1f19f/2

== system case6/AC_1/d_iq_load_5_block ==
  note: d_iq_load_5 in case6
      | $1121.6545740232\,\mathrm{vq}_{\mathrm{bus},5}-1094.814270933\,\mathrm{iq}_{\mathrm{load},5}-376.991118430775\,\mathrm{id}_{\mathrm{load},5}$
      | Automatically generated on 2025-10-31 19:20:40 .
  State_id_load_5_9ad4e : Inport
  State_iq_load_5_32b90 : Inport  Port=2
  State_vq_bus_5_ba55a : Inport  Port=3
  Add_d2919 : Sum
  Constant_-376.991118430775_54311 : Constant  Value=-376.991118430775
  Constant_1094.814270933_375a8 : Constant  Value=1094.814270933
  Constant_1121.6545740232_1df4f : Constant  Value=1121.6545740232
  Product_507b5 : Product
  Product_8dc3b : Product
  Product_a50a9 : Product
  Subtract_7cd7c : Sum  Inputs=+-
  Blockout_d_iq_load_5_d983c : Outport
  wires:
  Constant_-376.991118430775_54311/1 -> Product_8dc3b/1
  Product_507b5/1 -> Subtract_7cd7c/2
  State_id_load_5_9ad4e/1 -> Product_8dc3b/2
  Constant_1094.814270933_375a8/1 -> Product_507b5/1
  Product_8dc3b/1 -> Subtract_7cd7c/1
  State_iq_load_5_32b90/1 -> Product_507b5/2
  Constant_1121.6545740232_1df4f/1 -> Product_a50a9/1
  State_vq_bus_5_ba55a/1 -> Product_a50a9/2
  Subtract_7cd7c/1 -> Add_d2919/1
  Product_a50a9/1 -> Add_d2919/2
  Add_d2919/1 -> Blockout_d_iq_load_5_d983c/1

== system case6/AC_1/d_iq_load_7_block ==
  note: d_iq_load_7 in case6
      | $1171.3449213978\,\mathrm{vq}_{\mathrm{bus},7}-1042.68025815291\,\mathrm{iq}_{\mathrm{load},7}-376.991118430775\,\mathrm{id}_{\mathrm{load},7}$
      | Automatically generated on 2025-10-31 19:20:43 .
  State_id_load_7_34556 : Inport
  State_iq_load_7_eeef1 : Inport  Port=2
  State_vq_bus_7_dcb87 : Inport  Port=3
  Add_73887 : Sum
  Constant_-376.991118430775_e860b : Constant  Value=-376.991118430775
  Constant_1042.68025815291_15100 : Constant  Value=1042.68025815291
  Constant_1171.3449213978_60961 : Constant  Value=1171.3449213978
  Product_194da : Product
  Product_9b7bf : Product
  Product_e4326 : Product
  Subtract_2ca56 : Sum  Inputs=+-
  Blockout_d_iq_load_7_ba6b6 : Outport
  wires:
  Constant_-376.991118430775_e860b/1 -> Product_e4326/1
  Product_9b7bf/1 -> Subtract_2ca56/2
  State_id_load_7_34556/1 -> Product_e4326/2
  Constant_1042.68025815291_15100/1 -> Product_9b7bf/1
  Product_e4326/1 -> Subtract_2ca56/1
  State_iq_load_7_eeef1/1 -> Product_9b7bf/2
  Constant_1171.3449213978_60961/1 -> Product_194da/1
  State_vq_bus_7_dcb87/1 -> Product_194da/2
  Subtract_2ca56/1 -> Add_73887/1
  Product_194da/1 -> Add_73887/2
  Add_73887/1 -> Blockout_d_iq_load_7_ba6b6/1

== system case6/AC_1/d_iq_load_9_block ==
  note: d_iq_load_9 in case6
      | $1407.02236836831\,\mathrm{vq}_{\mathrm{bus},9}-912.345225962008\,\mathrm{iq}_{\mathrm{load},9}-376.991118430775\,\mathrm{id}_{\mathrm{load},9}$
      | Automatically generated on 2025-10-31 19:20:45 .
  State_id_load_9_30bf6 : Inport
  State_iq_load_9_4ab62 : Inport  Port=2
  State_vq_bus_9_7d406 : Inport  Port=3
  Add_676a0 : Sum
  Constant_-376.991118430775_aa1eb : Constant  Value=-376.991118430775
  Constant_1407.02236836831_4aea9 : Constant  Value=1407.02236836831
  Constant_912.345225962008_330f8 : Constant  Value=912.345225962008
  Product_a9e8b : Product
  Product_b8b7d : Product
  Product_ee45e : Product
  Subtract_1f04e : Sum  Inputs=+-
  Blockout_d_iq_load_9_4ac07 : Outport
  wires:
  Constant_-376.991118430775_aa1eb/1 -> Product_a9e8b/1
  Product_b8b7d/1 -> Subtract_1f04e/2
  State_id_load_9_30bf6/1 -> Product_a9e8b/2
  Add_676a0/1 -> Blockout_d_iq_load_9_4ac07/1
  Constant_912.345225962008_330f8/1 -> Product_b8b7d/1
  Product_ee45e/1 -> Add_676a0/2
  Product_a9e8b/1 -> Subtract_1f04e/1
  State_iq_load_9_4ab62/1 -> Product_b8b7d/2
  Constant_1407.02236836831_4aea9/1 -> Product_ee45e/1
  State_vq_bus_9_7d406/1 -> Product_ee45e/2
  Subtract_1f04e/1 -> Add_676a0/1

== system case6/AC_1/d_vd_bus_1_block ==
  note: d_vd_bus_1 in case6
      | $37699111.8430775\,\mathrm{id}_{\mathrm{bus},1}+376.991118430775\,\mathrm{vq}_{\mathrm{bus},1}$
      | Automatically generated on 2025-10-31 19:20:25 .
  Alge_id_bus_1_00dd9 : Inport
  State_vq_bus_1_7fdf6 : Inport  Port=2
  Add_da96b : Sum
  Constant_376.991118430775_6992a : Constant  Value=376.991118430775
  Constant_37699111.8430775_8184e : Constant  Value=37699111.8430775
  Product_0df35 : Product
  Product_ff1ea : Product
  Blockout_d_vd_bus_1_44375 : Outport
  wires:
  Constant_37699111.8430775_8184e/1 -> Product_ff1ea/1
  Product_0df35/1 -> Add_da96b/2
  Alge_id_bus_1_00dd9/1 -> Product_ff1ea/2
  Constant_376.991118430775_6992a/1 -> Product_0df35/1
  State_vq_bus_1_7fdf6/1 -> Product_0df35/2
  Add_da96b/1 -> Blockout_d_vd_bus_1_44375/1
  Product_ff1ea/1 -> Add_da96b/1

== system case6/AC_1/d_vd_bus_2_block ==
  note: d_vd_bus_2 in case6
      | $37699111.8430775\,\mathrm{id}_{\mathrm{bus},2}+376.991118430775\,\mathrm{vq}_{\mathrm{bus},2}$
      | Automatically generated on 2025-10-31 19:20:26 .
  Alge_id_bus_2_89ef1 : Inport
  State_vq_bus_2_41626 : Inport  Port=2
  Add_9cb81 : Sum
  Constant_376.991118430775_37c9e : Constant  Value=376.991118430775
  Constant_37699111.8430775_e9299 : Constant  Value=37699111.8430775
  Product_58dff : Product
  Product_e3d0b : Product
  Blockout_d_vd_bus_2_407e5 : Outport
  wires:
  Constant_37699111.8430775_e9299/1 -> Product_58dff/1
  Product_e3d0b/1 -> Add_9cb81/2
  Alge_id_bus_2_89ef1/1 -> Product_58dff/2
  Constant_376.991118430775_37c9e/1 -> Product_e3d0b/1
  Product_58dff/1 -> Add_9cb81/1
  State_vq_bus_2_41626/1 -> Product_e3d0b/2
  Add_9cb81/1 -> Blockout_d_vd_bus_2_407e5/1

== system case6/AC_1/d_vd_bus_3_block ==
  note: d_vd_bus_3 in case6
      | $37699111.8430775\,\mathrm{id}_{\mathrm{bus},3}+376.991118430775\,\mathrm{vq}_{\mathrm{bus},3}$
      | Automatically generated on 2025-10-31 19:20:27 .
  Alge_id_bus_3_d4dbd : Inport
  State_vq_bus_3_8d253 : Inport  Port=2
  Add_9db22 : Sum
  Constant_376.991118430775_6d8db : Constant  Value=376.991118430775
  Constant_37699111.8430775_791ee : Constant  Value=37699111.8430775
  Product_06984 : Product
  Product_a3f8d : Product
  Blockout_d_vd_bus_3_bca86 : Outport
  wires:
  Constant_37699111.8430775_791ee/1 -> Product_06984/1
  Product_a3f8d/1 -> Add_9db22/2
  Alge_id_bus_3_d4dbd/1 -> Product_06984/2
  Constant_376.991118430775_6d8db/1 -> Product_a3f8d/1
  Product_06984/1 -> Add_9db22/1
  State_vq_bus_3_8d253/1 -> Product_a3f8d/2
  Add_9db22/1 -> Blockout_d_vd_bus_3_bca86/1

== system case6/AC_1/d_vd_bus_4_block ==
  note: d_vd_bus_4 in case6
      | $2257.43184689087\,\mathrm{id}_{\mathrm{bus},4}+376.991118430775\,\mathrm{vq}_{\mathrm{bus},4}$
      | Automatically generated on 2025-10-31 19:20:27 .
  Alge_id_bus_4_6035c : Inport
  State_vq_bus_4_3285c : Inport  Port=2
  Add_7eb52 : Sum
  Constant_2257.43184689087_7f19c : Constant  Value=2257.43184689087
  Constant_376.991118430775_1ca63 : Constant  Value=376.991118430775
  Product_7968d : Product
  Product_8598b : Product
  Blockout_d_vd_bus_4_26ea1 : Outport
  wires:
  Constant_2257.43184689087_7f19c/1 -> Product_7968d/1
  Product_8598b/1 -> Add_7eb52/2
  Alge_id_bus_4_6035c/1 -> Product_7968d/2
  Constant_376.991118430775_1ca63/1 -> Product_8598b/1
  Product_7968d/1 -> Add_7eb52/1
  State_vq_bus_4_3285c/1 -> Product_8598b/2
  Add_7eb52/1 -> Blockout_d_vd_bus_4_26ea1/1

== system case6/AC_1/d_vd_bus_5_block ==
  note: d_vd_bus_5 in case6
      | $1461.2058853906\,\mathrm{id}_{\mathrm{bus},5}+376.991118430775\,\mathrm{vq}_{\mathrm{bus},5}$
      | Automatically generated on 2025-10-31 19:20:28 .
  Alge_id_bus_5_023a2 : Inport
  State_vq_bus_5_7e9fd : Inport  Port=2
  Add_48ccb : Sum
  Constant_1461.2058853906_b1867 : Constant  Value=1461.2058853906
  Constant_376.991118430775_8634e : Constant  Value=376.991118430775
  Product_6dfac : Product
  Product_90883 : Product
  Blockout_d_vd_bus_5_60ea3 : Outport
  wires:
  Constant_1461.2058853906_b1867/1 -> Product_90883/1
  Product_6dfac/1 -> Add_48ccb/2
  Alge_id_bus_5_023a2/1 -> Product_90883/2
  Constant_376.991118430775_8634e/1 -> Product_6dfac/1
  Product_90883/1 -> Add_48ccb/1
  State_vq_bus_5_7e9fd/1 -> Product_6dfac/2
  Add_48ccb/1 -> Blockout_d_vd_bus_5_60ea3/1

== system case6/AC_1/d_vd_bus_6_block ==
  note: d_vd_bus_6 in case6
      | $1329.77466818616\,\mathrm{id}_{\mathrm{bus},6}+376.991118430775\,\mathrm{vq}_{\mathrm{bus},6}$
      | Automatically generated on 2025-10-31 19:20:30 .
  Alge_id_bus_6_9129d : Inport
  State_vq_bus_6_48ab1 : Inport  Port=2
  Add_c4794 : Sum
  Constant_1329.77466818616_2cc60 : Constant  Value=1329.77466818616
  Constant_376.991118430775_6b1af : Constant  Value=376.991118430775
  Product_43b1f : Product
  Product_70eae : Product
  Blockout_d_vd_bus_6_93c4a : Outport
  wires:
  Constant_1329.77466818616_2cc60/1 -> Product_43b1f/1
  Product_70eae/1 -> Add_c4794/2
  Alge_id_bus_6_9129d/1 -> Product_43b1f/2
  Constant_376.991118430775_6b1af/1 -> Product_70eae/1
  Product_43b1f/1 -> Add_c4794/1
  State_vq_bus_6_48ab1/1 -> Product_70eae/2
  Add_c4794/1 -> Blockout_d_vd_bus_6_93c4a/1

== system case6/AC_1/d_vd_bus_7_block ==
  note: d_vd_bus_7 in case6
      | $2106.09563369148\,\mathrm{id}_{\mathrm{bus},7}+376.991118430775\,\mathrm{vq}_{\mathrm{bus},7}$
      | Automatically generated on 2025-10-31 19:20:32 .
  Alge_id_bus_7_e9afc : Inport
  State_vq_bus_7_f5bf3 : Inport  Port=2
  Add_6d183 : Sum
  Constant_2106.09563369148_ae832 : Constant  Value=2106.09563369148
  Constant_376.991118430775_da93a : Constant  Value=376.991118430775
  Product_09e68 : Product
  Product_f4cdc : Product
  Blockout_d_vd_bus_7_71af8 : Outport
  wires:
  Constant_2106.09563369148_ae832/1 -> Product_09e68/1
  Product_f4cdc/1 -> Add_6d183/2
  Alge_id_bus_7_e9afc/1 -> Product_09e68/2
  Constant_376.991118430775_da93a/1 -> Product_f4cdc/1
  Product_09e68/1 -> Add_6d183/1
  State_vq_bus_7_f5bf3/1 -> Product_f4cdc/2
  Add_6d183/1 -> Blockout_d_vd_bus_7_71af8/1

== system case6/AC_1/d_vd_bus_8_block ==
  note: d_vd_bus_8 in case6
      | $1657.10381727813\,\mathrm{id}_{\mathrm{bus},8}+376.991118430775\,\mathrm{vq}_{\mathrm{bus},8}$
      | Automatically generated on 2025-10-31 19:20:34 .
  Alge_id_bus_8_0f2fd : Inport
  State_vq_bus_8_543f2 : Inport  Port=2
  Add_c6b0d : Sum
  Constant_1657.10381727813_37fcd : Constant  Value=1657.10381727813
  Constant_376.991118430775_9d77c : Constant  Value=376.991118430775
  Product_db9bc : Product
  Product_f7331 : Product
  Blockout_d_vd_bus_8_ec3c4 : Outport
  wires:
  Constant_1657.10381727813_37fcd/1 -> Product_db9bc/1
  Product_f7331/1 -> Add_c6b0d/2
  Alge_id_bus_8_0f2fd/1 -> Product_db9bc/2
  Constant_376.991118430775_9d77c/1 -> Product_f7331/1
  Product_db9bc/1 -> Add_c6b0d/1
  State_vq_bus_8_543f2/1 -> Product_f7331/2
  Add_c6b0d/1 -> Blockout_d_vd_bus_8_ec3c4/1

== system case6/AC_1/d_vd_bus_9_block ==
  note: d_vd_bus_9 in case6
      | $1564.27849971276\,\mathrm{id}_{\mathrm{bus},9}+376.991118430775\,\mathrm{vq}_{\mathrm{bus},9}$
      | Automatically generated on 2025-10-31 19:20:36 .
  Alge_id_bus_9_39a0e : Inport
  State_vq_bus_9_da3ae : Inport  Port=2
  Add_49984 : Sum
  Constant_1564.27849971276_bb593 : Constant  Value=1564.27849971276
  Constant_376.991118430775_20641 : Constant  Value=376.991118430775
  Product_57be8 : Product
  Product_b584f : Product
  Blockout_d_vd_bus_9_20840 : Outport
  wires:
  Constant_1564.27849971276_bb593/1 -> Product_b584f/1
  Product_57be8/1 -> Add_49984/2
  Alge_id_bus_9_39a0e/1 -> Product_b584f/2
  Constant_376.991118430775_20641/1 -> Product_57be8/1
  Product_b584f/1 -> Add_49984/1
  State_vq_bus_9_da3ae/1 -> Product_57be8/2
  Add_49984/1 -> Blockout_d_vd_bus_9_20840/1

== system case6/AC_1/d_vq_bus_1_block ==
  note: d_vq_bus_1 in case6
      | $37699111.8430775\,\mathrm{iq}_{\mathrm{bus},1}-376.991118430775\,\mathrm{vd}_{\mathrm{bus},1}$
      | Automatically generated on 2025-10-31 19:20:26 .
  Alge_iq_bus_1_c2b12 : Inport
  State_vd_bus_1_7d44a : Inport  Port=2
  Constant_376.991118430775_e2ab4 : Constant  Value=376.991118430775
  Constant_37699111.8430775_83163 : Constant  Value=37699111.8430775
  Product_8baff : Product
  Product_af836 : Product
  Subtract_8e0b6 : Sum  Inputs=+-
  Blockout_d_vq_bus_1_24e4d : Outport
  wires:
  Constant_37699111.8430775_83163/1 -> Product_af836/1
  Constant_376.991118430775_e2ab4/1 -> Product_8baff/1
  Alge_iq_bus_1_c2b12/1 -> Product_af836/2
  State_vd_bus_1_7d44a/1 -> Product_8baff/2
  Product_af836/1 -> Subtract_8e0b6/1
  Product_8baff/1 -> Subtract_8e0b6/2
  Subtract_8e0b6/1 -> Blockout_d_vq_bus_1_24e4d/1

== system case6/AC_1/d_vq_bus_2_block ==
  note: d_vq_bus_2 in case6
      | $37699111.8430775\,\mathrm{iq}_{\mathrm{bus},2}-376.991118430775\,\mathrm{vd}_{\mathrm{bus},2}$
      | Automatically generated on 2025-10-31 19:20:26 .
  Alge_iq_bus_2_f979c : Inport
  State_vd_bus_2_661bf : Inport  Port=2
  Constant_376.991118430775_d4779 : Constant  Value=376.991118430775
  Constant_37699111.8430775_0a31b : Constant  Value=37699111.8430775
  Product_3adca : Product
  Product_c16fc : Product
  Subtract_f2425 : Sum  Inputs=+-
  Blockout_d_vq_bus_2_07cc4 : Outport
  wires:
  Constant_37699111.8430775_0a31b/1 -> Product_c16fc/1
  Constant_376.991118430775_d4779/1 -> Product_3adca/1
  Alge_iq_bus_2_f979c/1 -> Product_c16fc/2
  State_vd_bus_2_661bf/1 -> Product_3adca/2
  Product_c16fc/1 -> Subtract_f2425/1
  Product_3adca/1 -> Subtract_f2425/2
  Subtract_f2425/1 -> Blockout_d_vq_bus_2_07cc4/1

== system case6/AC_1/d_vq_bus_3_block ==
  note: d_vq_bus_3 in case6
      | $37699111.8430775\,\mathrm{iq}_{\mathrm{bus},3}-376.991118430775\,\mathrm{vd}_{\mathrm{bus},3}$
      | Automatically generated on 2025-10-31 19:20:27 .
  Alge_iq_bus_3_53990 : Inport
  State_vd_bus_3_f7b1a : Inport  Port=2
  Constant_376.991118430775_45269 : Constant  Value=376.991118430775
  Constant_37699111.8430775_1e3f8 : Constant  Value=37699111.8430775
  Product_21a83 : Product
  Product_3d59e : Product
  Subtract_70f8d : Sum  Inputs=+-
  Blockout_d_vq_bus_3_070a5 : Outport
  wires:
  Constant_37699111.8430775_1e3f8/1 -> Product_3d59e/1
  Constant_376.991118430775_45269/1 -> Product_21a83/1
  Alge_iq_bus_3_53990/1 -> Product_3d59e/2
  State_vd_bus_3_f7b1a/1 -> Product_21a83/2
  Product_3d59e/1 -> Subtract_70f8d/1
  Product_21a83/1 -> Subtract_70f8d/2
  Subtract_70f8d/1 -> Blockout_d_vq_bus_3_070a5/1

== system case6/AC_1/d_vq_bus_4_block ==
  note: d_vq_bus_4 in case6
      | $2257.43184689087\,\mathrm{iq}_{\mathrm{bus},4}-376.991118430775\,\mathrm{vd}_{\mathrm{bus},4}$
      | Automatically generated on 2025-10-31 19:20:27 .
  Alge_iq_bus_4_f3ad7 : Inport
  State_vd_bus_4_f40b6 : Inport  Port=2
  Constant_2257.43184689087_151a5 : Constant  Value=2257.43184689087
  Constant_376.991118430775_b2fdd : Constant  Value=376.991118430775
  Product_5ef4e : Product
  Product_d0588 : Product
  Subtract_24ea2 : Sum  Inputs=+-
  Blockout_d_vq_bus_4_5efd6 : Outport
  wires:
  Constant_2257.43184689087_151a5/1 -> Product_5ef4e/1
  Constant_376.991118430775_b2fdd/1 -> Product_d0588/1
  Alge_iq_bus_4_f3ad7/1 -> Product_5ef4e/2
  State_vd_bus_4_f40b6/1 -> Product_d0588/2
  Product_5ef4e/1 -> Subtract_24ea2/1
  Product_d0588/1 -> Subtract_24ea2/2
  Subtract_24ea2/1 -> Blockout_d_vq_bus_4_5efd6/1

== system case6/AC_1/d_vq_bus_5_block ==
  note: d_vq_bus_5 in case6
      | $1461.2058853906\,\mathrm{iq}_{\mathrm{bus},5}-376.991118430775\,\mathrm{vd}_{\mathrm{bus},5}$
      | Automatically generated on 2025-10-31 19:20:29 .
  Alge_iq_bus_5_9d80c : Inport
  State_vd_bus_5_a1a5e : Inport  Port=2
  Constant_1461.2058853906_1d7b8 : Constant  Value=1461.2058853906
  Constant_376.991118430775_b3170 : Constant  Value=376.991118430775
  Product_263cd : Product
  Product_bfe75 : Product
  Subtract_d2225 : Sum  Inputs=+-
  Blockout_d_vq_bus_5_a65b7 : Outport
  wires:
  Constant_1461.2058853906_1d7b8/1 -> Product_263cd/1
  Constant_376.991118430775_b3170/1 -> Product_bfe75/1
  Alge_iq_bus_5_9d80c/1 -> Product_263cd/2
  State_vd_bus_5_a1a5e/1 -> Product_bfe75/2
  Product_263cd/1 -> Subtract_d2225/1
  Product_bfe75/1 -> Subtract_d2225/2
  Subtract_d2225/1 -> Blockout_d_vq_bus_5_a65b7/1

== system case6/AC_1/d_vq_bus_6_block ==
  note: d_vq_bus_6 in case6
      | $1329.77466818616\,\mathrm{iq}_{\mathrm{bus},6}-376.991118430775\,\mathrm{vd}_{\mathrm{bus},6}$
      | Automatically generated on 2025-10-31 19:20:31 .
  Alge_iq_bus_6_37d1f : Inport
  State_vd_bus_6_8b156 : Inport  Port=2
  Constant_1329.77466818616_1a670 : Constant  Value=1329.77466818616
  Constant_376.991118430775_85dd2 : Constant  Value=376.991118430775
  Product_72e3c : Product
  Product_ab1e1 : Product
  Subtract_4fe23 : Sum  Inputs=+-
  Blockout_d_vq_bus_6_51bef : Outport
  wires:
  Constant_1329.77466818616_1a670/1 -> Product_72e3c/1
  Constant_376.991118430775_85dd2/1 -> Product_ab1e1/1
  Alge_iq_bus_6_37d1f/1 -> Product_72e3c/2
  State_vd_bus_6_8b156/1 -> Product_ab1e1/2
  Product_72e3c/1 -> Subtract_4fe23/1
  Product_ab1e1/1 -> Subtract_4fe23/2
  Subtract_4fe23/1 -> Blockout_d_vq_bus_6_51bef/1
